simulink model "fuzzyControl"  (R2015b)
settings: Solver=VariableStepAuto  StartTime=0.0  StopTime=10.0  RelTol=1e-3
libraries: fuzblock x1, simulink x1
settings Model: Creator=USER  LastModifiedBy=USER

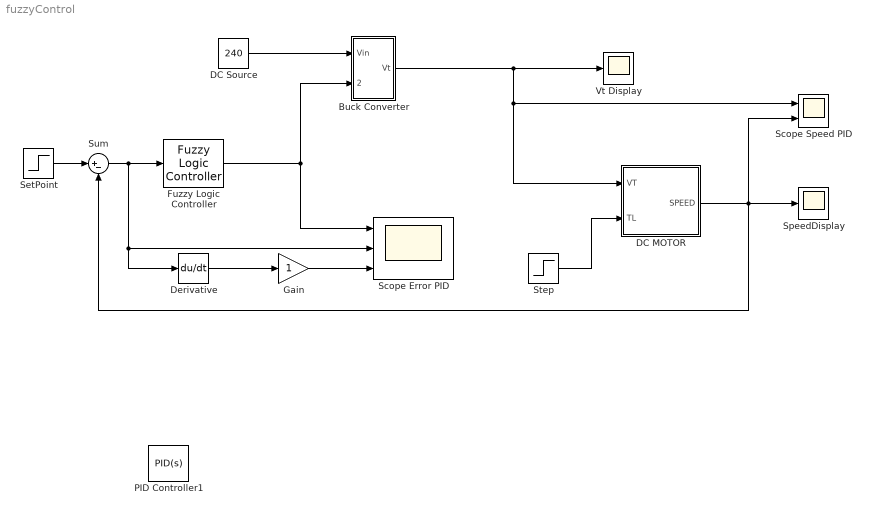
== system fuzzyControl ==
  Buck Converter : Subsystem
  DC MOTOR : Subsystem
  DC Source : Constant  Value=240
  Derivative : Derivative
  Fuzzy Logic Controller : fuzblock/Fuzzy Logic  Controller  fis=[]
  Gain : Gain
  PID Controller1 : simulink/Continuous/PID Controller  Controller=PID  TimeDomain=Continuous-time  SampleTime=-1  IntegratorMethod=Forward Euler  FilterMethod=Forward Euler  Form=Parallel  UseFilter=on  ControllerParametersSource=internal  P=0.01129  I=0.2911  D=0.0001084  N=6643  InitialConditionSource=internal  InitialConditionForIntegrator=0  InitialConditionForFilter=0  ExternalReset=none  LimitOutput=off  UpperSaturationLimit=inf  LowerSaturationLimit=-inf  LinearizeAsGain=on  AntiWindupMode=none  Kb=1  TrackingMode=off  Kt=1  PParamMin=[]  PParamMax=[]  IParamMin=[]  IParamMax=[]  DParamMin=[]  DParamMax=[]  NParamMin=[]  NParamMax=[]  KbParamMin=[]  KbParamMax=[]  KtParamMin=[]  KtParamMax=[]  POutMin=[]  POutMax=[]  IOutMin=[]  IOutMax=[]  DOutMin=[]  DOutMax=[]  NOutMin=[]  NOutMax=[]  KbOutMin=[]  KbOutMax=[]  KtOutMin=[]  KtOutMax=[]  IntegratorOutMin=[]  IntegratorOutMax=[]  FilterOutMin=[]  FilterOutMax=[]  SumOutMin=[]  SumOutMax=[]  SumI1OutMin=[]  SumI1OutMax=[]  SumI2OutMin=[]  SumI2OutMax=[]  SumI3OutMin=[]  SumI3OutMax=[]  SumDOutMin=[]  SumDOutMax=[]  SaturationOutMin=[]  SaturationOutMax=[]  IntegratorContinuousStateAttributes=''  IntegratorStateMustResolveToSignalObject=off  IntegratorRTWStateStorageClass=Auto  FilterContinuousStateAttributes=''  FilterStateMustResolveToSignalObject=off  FilterRTWStateStorageClass=Auto  DifferentiatorICPrevScaledInput=0  DifferentiatorOutMin=[]  DifferentiatorOutMax=[]
  Scope Error PID : Scope  NumInputPorts=3
  Scope Speed PID : Scope  NumInputPorts=2
  SetPoint : Step  SampleTime=0
  SpeedDisplay : Scope
  Step : Step  SampleTime=0
  Sum : Sum  Inputs=|+-
  Vt Display : Scope
  wires:
  Step/1 -> DC MOTOR/2(TL)
  DC MOTOR/1(SPEED) -> Sum/2, SpeedDisplay/1, Scope Speed PID/2
  Buck Converter/1(Vt) -> DC MOTOR/1(VT), Scope Speed PID/1, Vt Display/1
  Fuzzy Logic Controller/1 -> Scope Error PID/1, Buck Converter/2(Pwm)
  Sum/1 -> Fuzzy Logic Controller/1, Scope Error PID/2, Derivative/1
  SetPoint/1 -> Sum/1
  Derivative/1 -> Gain/1
  DC Source/1 -> Buck Converter/1(Vin)
  Gain/1 -> Scope Error PID/3

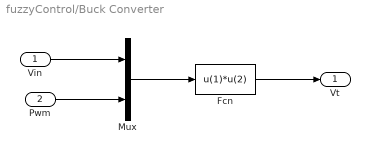
== system fuzzyControl/Buck Converter ==
  Vin : Inport
  Pwm : Inport  Port=2
  Fcn : Fcn  Expr=u(1)*u(2)
  Mux : Mux  Inputs=2
  Vt : Outport
  wires:
  Mux/1 -> Fcn/1
  Fcn/1 -> Vt/1
  Vin/1 -> Mux/1
  Pwm/1 -> Mux/2

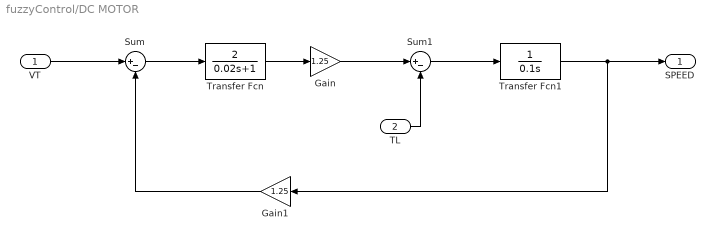
== system fuzzyControl/DC MOTOR ==
  VT : Inport
  TL : Inport  Port=2
  Gain : Gain  Gain=1.25
  Gain1 : Gain  Gain=1.25
  Sum : Sum  Inputs=|+-
  Sum1 : Sum  Inputs=|+-
  Transfer Fcn : TransferFcn  Numerator=[2]  Denominator=[0.02 1]
  Transfer Fcn1 : TransferFcn  Denominator=[0.1 0]
  SPEED : Outport
  wires:
  Transfer Fcn1/1 -> SPEED/1, Gain1/1
  Gain1/1 -> Sum/2
  Transfer Fcn/1 -> Gain/1
  VT/1 -> Sum/1
  Sum1/1 -> Transfer Fcn1/1
  TL/1 -> Sum1/2
  Gain/1 -> Sum1/1
  Sum/1 -> Transfer Fcn/1
